simulink model "pendulum_model_complete"  (R2024a)
settings: Solver=FixedStepAuto  StartTime=0.0  StopTime=10  FixedStep=Ts  RelTol=1e-3
values from neighbouring files (symbols this model uses):
  A = [0  1; -19.62  0]    [pendulum_parameters_complete.mat]
  B = [0 4]    [pendulum_parameters_complete.mat]
  C = [1 0]    [pendulum_parameters_complete.mat]
  D = 0    [pendulum_parameters_complete.mat]
  g = 9.81    [pendulum_parameters_complete.mat]
  KF_theta0 = 0.174532925199    [pendulum_parameters_complete.mat]
  KF_theta_dot0 = 0    [pendulum_parameters_complete.mat]
  L = 0.5    [pendulum_parameters_complete.mat]
  m = 1    [pendulum_parameters_complete.mat]
  R = 0.0001    [pendulum_parameters_complete.mat]
  theta0 = 0.174532925199    [pendulum_parameters_complete.mat]
  theta_dot0 = 0    [pendulum_parameters_complete.mat]
undefined symbols (not defined in the file or in its folder): Continuous, Time
libraries: simulink_extras x3, simulink x2, ctrlSharedLib x1
settings Model: Creator=mulusoy  LastModifiedBy=jantonio
settings DebuggingCC: UnconnectedInputMsg=warning  UnconnectedOutputMsg=warning  UnconnectedLineMsg=warning
settings ModelReferenceCC: EnableRefExpFcnMdlSchedulingChecks=on
settings RTWCC: GPUComputeCapability=3.5  DLArmComputeVersion=19.05
settings ExplorerConfigSet: SimMechanicsOpenEditorOnUpdate=off  InternalSimMechanicsExplorerSettings="<ExplorerConfiguration><canonicalview>planar_xy</canonicalview><AnimationSetting><BasePlaybackSpeed>1.0</BasePlaybackSpeed><PlaybackSpeedFactor>1.0</PlaybackSpeedFactor></AnimationSetting><TilePanel><TileInfo><Tiles Columns=\"1\" Count=\"1\" Rows=\"1\"><Column Weight=\"1\"/><Row Weight=\"1\"/><Tile Height=\"1\" Width=\"1\" X=\"0\" Y=\"0\"/></Tiles></TileInfo><SceneInfo><SceneViewer><BGColor><R>0.60000002384185791</R><G>0.60000002384185791</G><B>0.60000002384185791</B></BGColor><Camera><DoPerspective>off</DoPerspective><Position><X>-2.81337411700555151e-09</X><Y>-0.263610325606282447</Y><Z>1.00000001491760937</Z></Position><Center><X>-2.81337411700555151e-09</X><Y>-0.263610325606282447</Y><Z>1.49176093700020829e-08</Z></Center><Up><X>0</X><Y>1</Y><Z>0</Z></Up><ViewLimDist>1</ViewLimDist><YLim>0.297268618643283855</YLim><XLim>0.57836459223084502</XLim></Camera></SceneViewer></SceneInfo></TilePanel><MechEditorPanel><Cameras/><GfxPanelCameraMap/><VideoCreator><PlaybackSpeedRatio>1.0</PlaybackSpeedRatio><FrameRate>30</FrameRate><VideoFormat>Motion JPEG AVI</VideoFormat><FrameSize>auto</FrameSize></VideoCreator></MechEditorPanel></ExplorerConfiguration>"

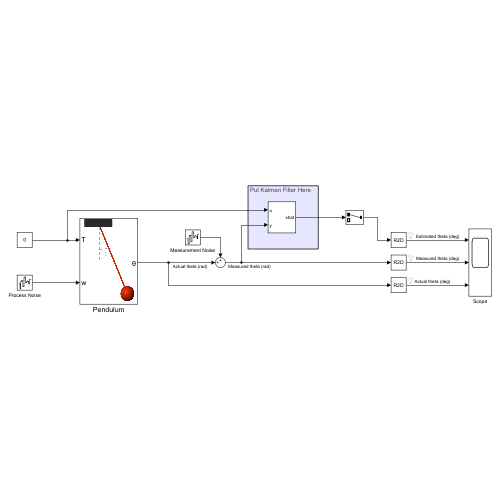
[thumbnail: Simulink's stored preview of the top-level diagram]
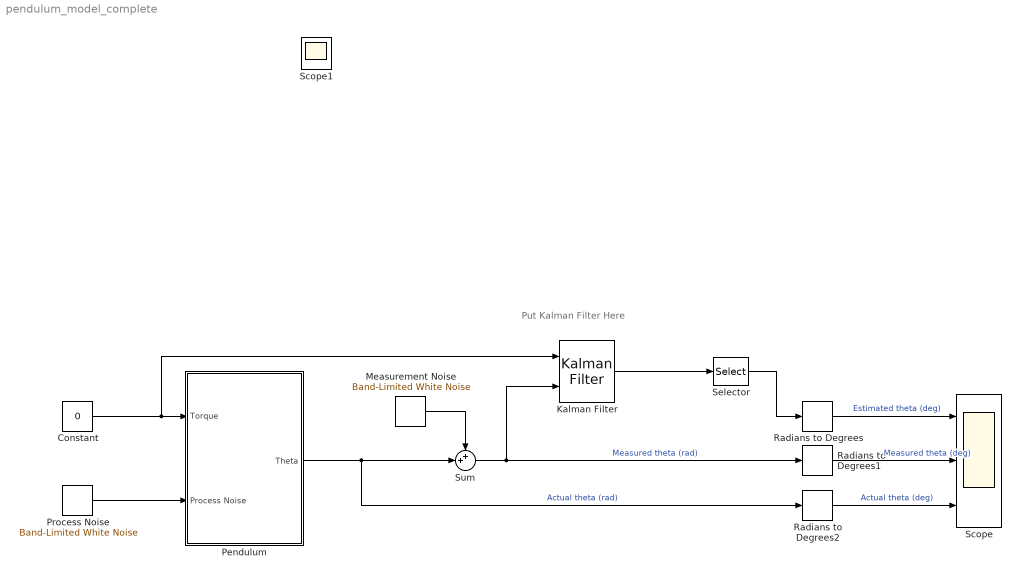
== system pendulum_model_complete ==
  note: Put Kalman Filter Here
  Constant : Constant  Value=0
  Kalman Filter : ctrlSharedLib/Kalman Filter  TimeDomain=Continuous-Time  UseCurrentEstimator=on  ModelSource=Individual A, B, C, D matrices  ModelSourceVariable=ss(0.95,1,1,0,1)  A=A  B=B  C=C  D=D  NumberOfStates=1  NumberOfInputs=1  NumberOfOutputs=1  InitialEstimateSource=Dialog  X0=[KF_theta0 KF_theta_dot0]  P0=10  UseK=off  UseGH=off  NumberOfProcessNoiseInputs=1  G=1  TimeInvariantG=on  H=0  TimeInvariantH=on  Q=Q  TimeInvariantQ=on  R=R  TimeInvariantR=on  N=0  TimeInvariantN=on  AddInputPort=on  AddEnablePort=off  OutputEstimatedY=off  OutputP=off  Ts=-1
  Measurement Noise : simulink/Sources/Band-Limited White Noise  Cov=1e-6  Ts=0.01  seed=[23341]
  Pendulum : Subsystem  mask{theta_0=theta0, theta_dot_0=theta_dot0}
      mask prompts: theta_0 "Initial value of theta"; theta_dot_0 "Initial value of theta_dot"
      mask Display:
      | image('pend.png');
      | port_label('input',1,'T');
      | port_label('input',2,'w');
      | port_label('output',1,'\theta','interpreter','tex');
  Process Noise : simulink/Sources/Band-Limited White Noise  Cov=w  Ts=0.01  seed=[23341]
  Radians to Degrees : simulink_extras/Transformations/Radians to Degrees
  Radians to Degrees1 : simulink_extras/Transformations/Radians to Degrees
  Radians to Degrees2 : simulink_extras/Transformations/Radians to Degrees
  Scope : Scope  NumInputPorts=3
  Selector : Selector  InputPortWidth=2  IndexOptions=Index vector (dialog)  Indices=1  OutputSizes=1
  Sum : Sum  Inputs=++|
  Scope1 : Scope
  wires:
  Measurement Noise/1 -> Sum/1
  Radians to Degrees1/1 -> Scope/2  "Measured theta (deg)"
  Pendulum/1(Theta) -> Radians to Degrees2/1, Sum/2  "Actual theta (rad)"
  Radians to Degrees2/1 -> Scope/3  "Actual theta (deg)"
  Constant/1 -> Kalman Filter/1, Pendulum/1(Torque)
  Process Noise/1 -> Pendulum/2(Process Noise)
  Selector/1 -> Radians to Degrees/1
  Sum/1 -> Kalman Filter/2, Radians to Degrees1/1  "Measured theta (rad)"
  Radians to Degrees/1 -> Scope/1  "Estimated theta (deg)"
  Kalman Filter/1 -> Selector/1

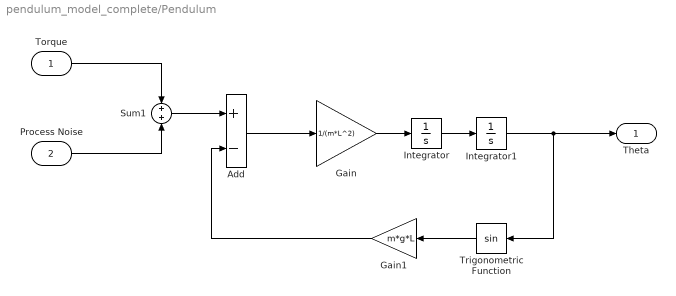
== system pendulum_model_complete/Pendulum ==
  Torque : Inport
  Process Noise : Inport  Port=2
  Add : Sum  Inputs=+-
  Gain : Gain  Gain=1/(m*L^2)
  Gain1 : Gain  Gain=m*g*L
  Integrator : Integrator  InitialCondition=theta_dot0
  Integrator1 : Integrator  InitialCondition=theta_0
      settings: AttributesFormatString=%<InitialCondition> rad
  Sum1 : Sum  Inputs=+|+
  Trigonometric Function : Trigonometry
  Theta : Outport
  wires:
  Torque/1 -> Sum1/1
  Process Noise/1 -> Sum1/2
  Sum1/1 -> Add/1
  Trigonometric Function/1 -> Gain1/1
  Gain1/1 -> Add/2
  Gain/1 -> Integrator/1
  Add/1 -> Gain/1
  Integrator/1 -> Integrator1/1
  Integrator1/1 -> Theta/1, Trigonometric Function/1
